simulink model "PIDmotor"  (R2015a)
settings: Solver=ode45  StartTime=0.0  StopTime=t_end  MaxStep=0.001  RelTol=1e-3
values from neighbouring files (symbols this model uses):
  b = 1*10^-3    (= 0.001)    [Simulation_script.m]
  delay = 0e-3    (= 0)    [Simulation_script.m]
  i = 14    [Simulation_script.m]
  I = 1.4    [Simulation_script.m]
  J = r^2*100/(i^2)    (= 0.00510204081633)    [Simulation_script.m]
  Ke = 0.147    [Simulation_script.m]
  Kt = 0.147    [Simulation_script.m]
  L = 0.82*10^-3    (= 0.00082)    [Simulation_script.m]
  P = 0.2    [Simulation_script.m]
  R = 1.03    [Simulation_script.m]
  r = 0.1    [Simulation_script.m]
  target_angular_velocity = 280    [Simulation_script.m]
settings Model: CovSFcnEnable=off  Creator=tlantela  LastModifiedBy=tlantela
settings DebuggingCC: SolverPrmCheckMsg=warning

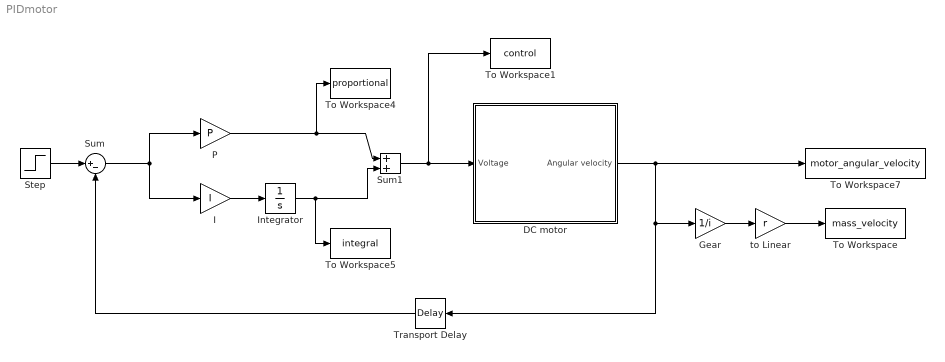
== system PIDmotor ==
  DC motor : Subsystem
  Gear : Gain  Gain=1/i
  I : Gain  Gain=I
  Integrator : Integrator
  P : Gain  Gain=P
  Step : Step  Time=0  After=target_angular_velocity  SampleTime=0
  Sum : Sum  Inputs=|+-
  Sum1 : Sum
  To Workspace : ToWorkspace  VariableName=mass_velocity  SaveFormat=Timeseries  SampleTime=-1
  To Workspace1 : ToWorkspace  VariableName=control  SaveFormat=Timeseries  SampleTime=-1
  To Workspace4 : ToWorkspace  VariableName=proportional  SaveFormat=Timeseries  SampleTime=-1
  To Workspace5 : ToWorkspace  VariableName=integral  SaveFormat=Timeseries  SampleTime=-1
  To Workspace7 : ToWorkspace  VariableName=motor_angular_velocity  SaveFormat=Timeseries  SampleTime=-1
  Transport Delay : TransportDelay  DelayTime=delay
  to Linear : Gain  Gain=r
  wires:
  Sum/1 -> I/1, P/1
  I/1 -> Integrator/1
  P/1 -> Sum1/1, To Workspace4/1
  Integrator/1 -> Sum1/2, To Workspace5/1
  Transport Delay/1 -> Sum/2
  DC motor/1(Angular velocity) -> Transport Delay/1, Gear/1, To Workspace7/1
  Step/1 -> Sum/1
  Sum1/1 -> DC motor/1(Voltage), To Workspace1/1
  Gear/1 -> to Linear/1
  to Linear/1 -> To Workspace/1

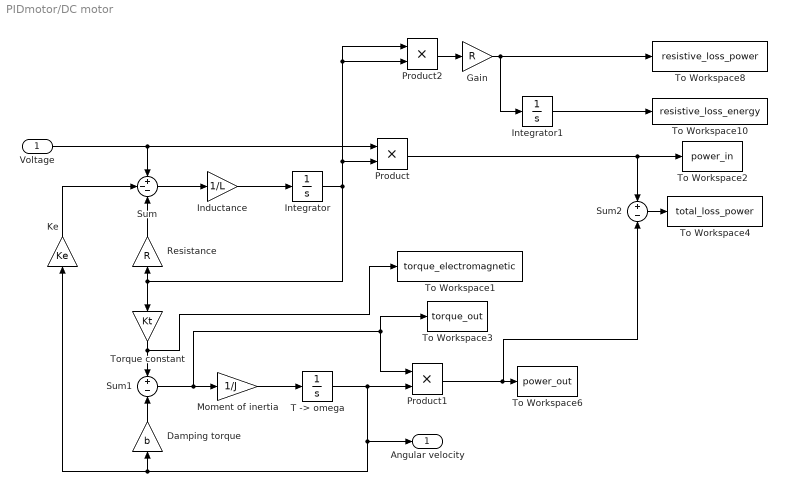
== system PIDmotor/DC motor ==
  Voltage : Inport
  Damping torque : Gain  Gain=b
  Gain : Gain  Gain=R
  Inductance : Gain  Gain=1/L
  Integrator : Integrator
  Integrator1 : Integrator
  Ke : Gain  Gain=Ke
  Moment of inertia : Gain  Gain=1/J
  Product : Product
  Product1 : Product
  Product2 : Product
  Resistance : Gain  Gain=R
  Sum : Sum  Inputs=+--
  Sum1 : Sum  Inputs=+-
  Sum2 : Sum  Inputs=+-
  "T -> omega" : Integrator
  To Workspace1 : ToWorkspace  VariableName=torque_electromagnetic  SaveFormat=Timeseries  SampleTime=-1
  To Workspace10 : ToWorkspace  VariableName=resistive_loss_energy  SaveFormat=Timeseries  SampleTime=-1
  To Workspace2 : ToWorkspace  VariableName=power_in  SaveFormat=Timeseries  SampleTime=-1
  To Workspace3 : ToWorkspace  VariableName=torque_out  SaveFormat=Timeseries  SampleTime=-1
  To Workspace4 : ToWorkspace  VariableName=total_loss_power  SaveFormat=Timeseries  SampleTime=-1
  To Workspace6 : ToWorkspace  VariableName=power_out  SaveFormat=Timeseries  SampleTime=-1
  To Workspace8 : ToWorkspace  VariableName=resistive_loss_power  SaveFormat=Timeseries  SampleTime=-1
  Torque constant : Gain  Gain=Kt
  Angular velocity : Outport
  wires:
  Voltage/1 -> Sum/1, Product/1
  Sum/1 -> Inductance/1
  Inductance/1 -> Integrator/1
  Integrator/1 -> Product2/1, Product2/2, Product/2, Torque constant/1, Resistance/1
  Ke/1 -> Sum/2
  Resistance/1 -> Sum/3
  Torque constant/1 -> To Workspace1/1, Sum1/1
  Moment of inertia/1 -> "T -> omega"/1
  Product/1 -> To Workspace2/1, Sum2/1
  Damping torque/1 -> Sum1/2
  Sum1/1 -> To Workspace3/1, Product1/1, Moment of inertia/1
  Product1/1 -> To Workspace6/1, Sum2/2
  "T -> omega"/1 -> Ke/1, Damping torque/1, Angular velocity/1, Product1/2
  Gain/1 -> Integrator1/1, To Workspace8/1
  Product2/1 -> Gain/1
  Integrator1/1 -> To Workspace10/1
  Sum2/1 -> To Workspace4/1
